simulink model "sgMdl_Serial_RS485Loopback"  (R2024b)
settings: Solver=FixedStepAuto  StartTime=0.0  StopTime=inf  RelTol=1e-3  EnableMultiTasking=on
undefined symbols (not defined in the file): standard
libraries: slrealtimeseriallib x16, speedgoatlib_serial x9
Description:
  | Serial - RS485 Loopback
settings Model: ModifiedByFormat=Speedgoat  Creator=Speedgoat  LastModifiedBy=Speedgoat
settings SolverCC: ConcurrentTasks=on  AlgebraicLoopSolver=TrustRegion  PositivePriorityOrder=on  InsertRTBMode=Never (minimum delay)
settings DataIOCC: LimitDataPoints=on  SaveFormat=Array  SignalLoggingSaveFormat=ModelDataLogs  ReturnWorkspaceOutputs=off
settings OptimizationCC: BlockReduction=off  OptimizeBlockIOStorage=off  BufferReuse=off  GlobalBufferReuse=off  ExpressionFolding=off  ExpressionDepthLimit=2147483647  LocalBlockOutputs=off  OptimizeDataStoreBuffers=off  BusAssignmentInplaceUpdate=off
settings DebuggingCC: UnderspecifiedInitializationDetection=Classic  MergeDetectMultiDrivingBlocksExec=none  SolverPrmCheckMsg=warning  TasksWithSamePriorityMsg=none  FcnCallInpInsideContextMsg=warning  StateNameClashWarn=warning  SFUnexpectedBacktrackingDiag=warning  SFNoUnconditionalDefaultTransitionDiag=warning  SFExecutionAtInitializationDiag=none  ArithmeticOperatorsInVariantConditions=warning
settings HardwareCC: ProdBitPerLong=64  ProdLongLongMode=on  ProdHWDeviceType=Intel->x86-64 (Linux 64)
settings ModelReferenceCC: EnableRefExpFcnMdlSchedulingChecks=on  PropagateSignalLabelsOutOfModel=off
settings SFSimCC: SimUseLocalCustomCode=off  CustomCodeUndefinedFunction=UseInterfaceOnly
settings RTWCC: Description=Speedgoat Real-Time Target Machine  SystemTargetFile=speedgoat.tlc  TemplateMakefile=slrealtime_default_tmf  RTWUseLocalCustomCode=off  Toolchain=Simulink Real-Time Toolchain  BuildConfiguration=Faster Runs  TargetLang=C++  GPUComputeCapability=3.5  DLArmComputeVersion=19.05
settings CodeAppCC: StateflowObjectComments=on
settings SimulinkRealTimeTargetCC: SubcomponentCodeInterfacePackaging=Reusable function  InstructionSetFMA=off  LogToMDFFile=off  SLRTFileLogMaxRuns=10  UseGCCFastMath=on
settings ConfigComp: CovMetricSettings=dw  CovSaveCumulativeToWorkspaceVar=on  CovSaveSingleToWorkspaceVar=on  CovExternalEMLEnable=off  CovSFcnEnable=off  CovBoundaryAbsTol=1.0e-5

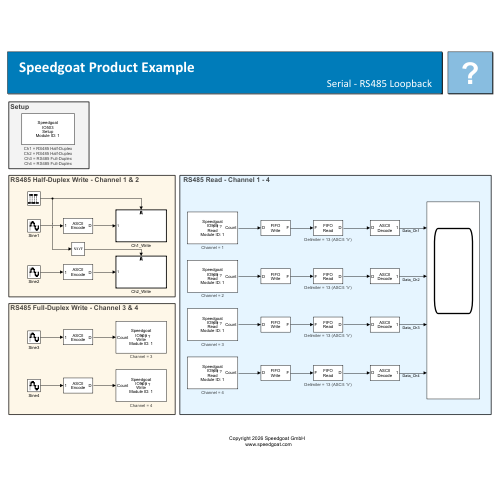
[thumbnail: Simulink's stored preview of the top-level diagram]
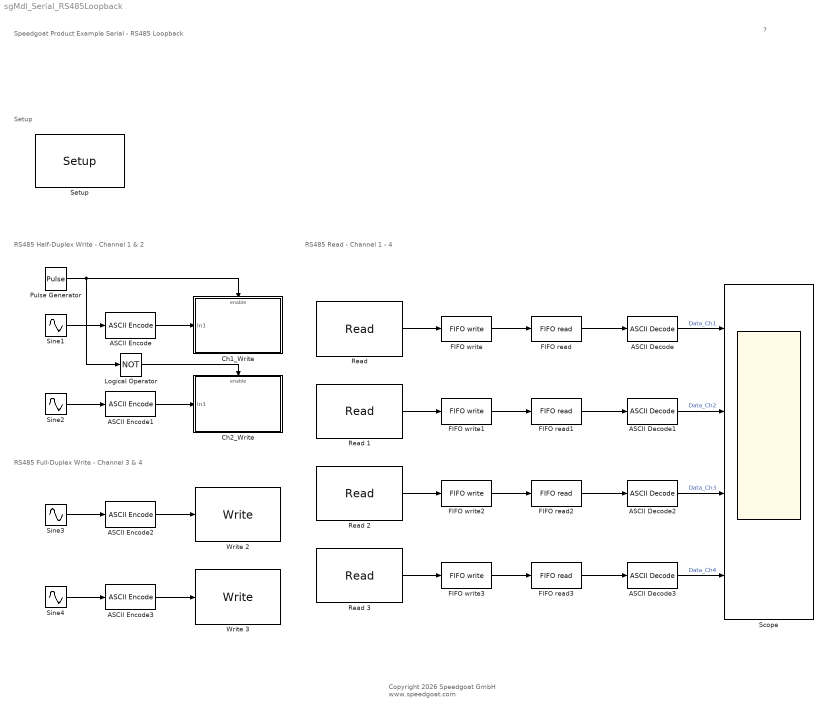
== system sgMdl_Serial_RS485Loopback ==
  note: RS485 Read - Channel 1 - 4
  note: RS485 Half-Duplex Write - Channel 1 & 2
  note: Setup
  note: RS485 Full-Duplex Write - Channel 3 & 4
  note: Speedgoat Product Example
      | Serial - RS485 Loopback
  note: ?
  note: Copyright 2026 Speedgoat GmbH
      |  www.speedgoat.com
  ASCII Decode{,1..3} (4 alike) : slrealtimeseriallib/ASCII Decode  format=%f\r  nvars=1  vartypes={'double'}
  ASCII Encode{,1..3} (4 alike) : slrealtimeseriallib/ASCII Encode  format=%f\r  nvars=1  maxlength=64  vartypes={ 'double' }
  Ch1_Write : Subsystem  TreatAsAtomicUnit=on
  Ch2_Write : Subsystem  TreatAsAtomicUnit=on
  FIFO read{,1..3} (4 alike) : slrealtimeseriallib/FIFO read  maxsize=128  minsize=1  usedelimiter=on  delimiter=13  outputtype=8 bit uint null terminated  enable=off  enableout=off  sampletime=0.01
      settings: AttributesFormatString=Delimiter = %<delimiter> (ASCII: '\r')
  FIFO write : slrealtimeseriallib/FIFO write  size=128  inputtype=8 bit uint null terminated  present=off  sampletime=-1  id=Rx Ch1 overflow
  FIFO write1 : slrealtimeseriallib/FIFO write  size=128  inputtype=8 bit uint null terminated  present=off  sampletime=-1  id=Rx Ch2 overflow
  FIFO write2 : slrealtimeseriallib/FIFO write  size=128  inputtype=8 bit uint null terminated  present=off  sampletime=-1  id=Rx Ch3 overflow
  FIFO write3 : slrealtimeseriallib/FIFO write  size=128  inputtype=8 bit uint null terminated  present=off  sampletime=-1  id=Rx Ch4 overflow
  Logical Operator : Logic  Operator=NOT  AllPortsSameDT=off  OutDataTypeStr=boolean
  Pulse Generator : DiscretePulseGenerator  SampleTime=0.01
  "Read " : speedgoatlib_serial/Speedgoat Shared blocks/Read   parModuleType=IO503  parModuleId=1  parChannel=1  parSampleTime=0.01  parFlush=on  parEnLegacy=on  parDataType=8 bit uint null terminated  parSlot=-1  parRxSwFifoSize=64
      settings: AttributesFormatString=Channel = %<parChannel>
  Read 1 : speedgoatlib_serial/Speedgoat Shared blocks/Read   parModuleType=IO503  parModuleId=1  parChannel=2  parSampleTime=0.01  parFlush=on  parEnLegacy=on  parDataType=8 bit uint null terminated  parSlot=-1  parRxSwFifoSize=64
      settings: AttributesFormatString=Channel = %<parChannel>
  Read 2 : speedgoatlib_serial/Speedgoat Shared blocks/Read   parModuleType=IO503  parModuleId=1  parChannel=3  parSampleTime=0.01  parFlush=on  parEnLegacy=on  parDataType=8 bit uint null terminated  parSlot=-1  parRxSwFifoSize=64
      settings: AttributesFormatString=Channel = %<parChannel>
  Read 3 : speedgoatlib_serial/Speedgoat Shared blocks/Read   parModuleType=IO503  parModuleId=1  parChannel=4  parSampleTime=0.01  parFlush=on  parEnLegacy=on  parDataType=8 bit uint null terminated  parSlot=-1  parRxSwFifoSize=64
      settings: AttributesFormatString=Channel = %<parChannel>
  Scope : Scope  NumInputPorts=4
  "Setup " : speedgoatlib_serial/Speedgoat Shared blocks/Setup   parModuleType=IO503  parModuleId=1  parSlot=-1  parOscillator=44.2368  parOscillator581=125  parTransceiver1=RS485 Half-Duplex  parTransceiver2=RS485 Half-Duplex  parTransceiver3=RS485 Full-Duplex  parTransceiver4=RS485 Full-Duplex  parTransceiver5=Disabled  parTransceiver6=Disabled  parTransceiver7=Disabled  parTransceiver8=Disabled  parTxTerm1=on  parRxTerm1=off  parMessageMonitoring1=off  parAutoTurnaround1=off  parTurnaroundDelay1=0  parStandardBaud1=on  parBaudrate1=2764800  parBaudDivisor1=1  parSamplingRate1=16x (standard)  parPrescale1=None  parCalcBaud1=2764800  parParity1=None  parDataBits1=8  parStopBits1=1  parTxTrigLvl1=1  parRxTrigLvl1=8  parHandshake1=none  parRtsHysteresis1=0  parXon1=17  parXoff1=19  parTxSwFifoSize1=64  parRxSwFifoSize1=64  parTxTerm2=on  parRxTerm2=off  parMessageMonitoring2=off  parAutoTurnaround2=off  parTurnaroundDelay2=0  parStandardBaud2=on  parBaudrate2=2764800  parBaudDivisor2=1  parSamplingRate2=16x (standard)  parPrescale2=None  parCalcBaud2=2764800  parParity2=None  parDataBits2=8  parStopBits2=1  parTxTrigLvl2=1  parRxTrigLvl2=8  parHandshake2=none  parRtsHysteresis2=0  parXon2=17  parXoff2=19  parTxSwFifoSize2=64  parRxSwFifoSize2=64  parTxTerm3=on  parRxTerm3=on  parMessageMonitoring3=off  parAutoTurnaround3=off  parTurnaroundDelay3=0  parStandardBaud3=on  parBaudrate3=2764800  parBaudDivisor3=1  parSamplingRate3=16x (standard)  parPrescale3=None  parCalcBaud3=2764800  parParity3=None  parDataBits3=8  parStopBits3=1  parTxTrigLvl3=1  parRxTrigLvl3=8  parHandshake3=none  parRtsHysteresis3=0  parXon3=17  parXoff3=19  parTxSwFifoSize3=64  parRxSwFifoSize3=64  parTxTerm4=on  parRxTerm4=on  parMessageMonitoring4=off  parAutoTurnaround4=off  parTurnaroundDelay4=0  parStandardBaud4=on  parBaudrate4=2764800  parBaudDivisor4=1  parSamplingRate4=16x (standard)  parPrescale4=None  parCalcBaud4=2764800  parParity4=None  parDataBits4=8  parStopBits4=1  parTxTrigLvl4=1  parRxTrigLvl4=8  parHandshake4=none  parRtsHysteresis4=0  parXon4=17  parXoff4=19  parTxSwFifoSize4=64  parRxSwFifoSize4=64  parTxTerm5=off  parRxTerm5=off  parMessageMonitoring5=off  parAutoTurnaround5=off  parTurnaroundDelay5=0  parStandardBaud5=on  parBaudrate5=115200  parBaudDivisor5=1  parSamplingRate5=16x (standard)  parPrescale5=None  parCalcBaud5=2764800  parParity5=None  parDataBits5=8  parStopBits5=1  parTxTrigLvl5=1  parRxTrigLvl5=1  parHandshake5=none  parRtsHysteresis5=0  parXon5=17  parXoff5=19  parTxSwFifoSize5=1024  parRxSwFifoSize5=1024  parTxTerm6=off  parRxTerm6=off  parMessageMonitoring6=off  parAutoTurnaround6=off  parTurnaroundDelay6=0  parStandardBaud6=on  parBaudrate6=115200  parBaudDivisor6=1  parSamplingRate6=16x (standard)  parPrescale6=None  parCalcBaud6=2764800  parParity6=None  parDataBits6=8  parStopBits6=1  parTxTrigLvl6=1  parRxTrigLvl6=1  parHandshake6=none  parRtsHysteresis6=0  parXon6=17  parXoff6=19  parTxSwFifoSize6=1024  parRxSwFifoSize6=1024  parTxTerm7=off  parRxTerm7=off  parMessageMonitoring7=off  parAutoTurnaround7=off  parTurnaroundDelay7=0  parStandardBaud7=on  parBaudrate7=115200  parBaudDivisor7=1  parSamplingRate7=16x (standard)  parPrescale7=None  parCalcBaud7=2764800  parParity7=None  parDataBits7=8  parStopBits7=1  parTxTrigLvl7=1  parRxTrigLvl7=1  parHandshake7=none  parRtsHysteresis7=0  parXon7=17  parXoff7=19  parTxSwFifoSize7=1024  parRxSwFifoSize7=1024  parTxTerm8=off  parRxTerm8=off  parMessageMonitoring8=off  parAutoTurnaround8=off  parTurnaroundDelay8=0  parStandardBaud8=on  parBaudrate8=115200  parBaudDivisor8=1  parSamplingRate8=16x (standard)  parPrescale8=None  parCalcBaud8=2764800  parParity8=None  parDataBits8=8  parStopBits8=1  parTxTrigLvl8=1  parRxTrigLvl8=1  parHandshake8=none  parRtsHysteresis8=0  parXon8=17  parXoff8=19  parTxSwFifoSize8=1024  parRxSwFifoSize8=1024
      settings: SourceProductName=Simulink Real-Time: Speedgoat I/O Driver Library
      settings: AttributesFormatString=|
      | Ch1 = %<parTransceiver1>
      | Ch2 = %<parTransceiver2>
      | Ch3 = %<parTransceiver3>
      | Ch4 = %<parTransceiver4>
  Sine1 : Sin  Amplitude=10  Bias=127  Frequency=1*2*pi  SampleTime=0.01
  Sine2 : Sin  Amplitude=20  Bias=127  Frequency=1*2*pi  SampleTime=0.01
  Sine3 : Sin  Amplitude=30  Bias=127  Frequency=1*2*pi  SampleTime=0.01
  Sine4 : Sin  Amplitude=40  Bias=127  Frequency=1*2*pi  SampleTime=0.01
  Write 2 : speedgoatlib_serial/Speedgoat Shared blocks/Write   parModuleType=IO503  parModuleId=1  parChannel=3  parSampleTime=-1  parEnLegacy=on  parDataType=8 bit uint null terminated  parMdlStopMsgEnable=off  parMdlStopMsgData=['CONF' char(13)]  parMdlStopFifoOptions=Write to TX FIFO directly  parMdlStopMsgsDataArr=[67 79 78 70 13]  parMdlStopMsgsDataSize=5  parSlot=-1  parTxSwFifoSize=64
      settings: AttributesFormatString=Channel = %<parChannel>
  Write 3 : speedgoatlib_serial/Speedgoat Shared blocks/Write   parModuleType=IO503  parModuleId=1  parChannel=4  parSampleTime=-1  parEnLegacy=on  parDataType=8 bit uint null terminated  parMdlStopMsgEnable=off  parMdlStopMsgData=['CONF' char(13)]  parMdlStopFifoOptions=Write to TX FIFO directly  parMdlStopMsgsDataArr=[67 79 78 70 13]  parMdlStopMsgsDataSize=5  parSlot=-1  parTxSwFifoSize=64
      settings: AttributesFormatString=Channel = %<parChannel>
  wires:
  Sine4/1 -> ASCII Encode3/1
  Sine3/1 -> ASCII Encode2/1
  ASCII Decode/1 -> Scope/1  "Data_Ch1"
  ASCII Decode1/1 -> Scope/2  "Data_Ch2"
  ASCII Decode2/1 -> Scope/3  "Data_Ch3"
  ASCII Decode3/1 -> Scope/4  "Data_Ch4"
  FIFO write/1 -> FIFO read/1
  "Read "/1 -> FIFO write/1
  FIFO write1/1 -> FIFO read1/1
  Read 1/1 -> FIFO write1/1
  FIFO write2/1 -> FIFO read2/1
  FIFO write3/1 -> FIFO read3/1
  FIFO read1/1 -> ASCII Decode1/1
  FIFO read2/1 -> ASCII Decode2/1
  FIFO read3/1 -> ASCII Decode3/1
  Read 2/1 -> FIFO write2/1
  Read 3/1 -> FIFO write3/1
  FIFO read/1 -> ASCII Decode/1
  ASCII Encode2/1 -> Write 2/1
  ASCII Encode3/1 -> Write 3/1
  Pulse Generator/1 -> Ch1_Write/Enable, Logical Operator/1
  Logical Operator/1 -> Ch2_Write/Enable
  Sine1/1 -> ASCII Encode/1
  ASCII Encode/1 -> Ch1_Write/1(In1)
  Sine2/1 -> ASCII Encode1/1
  ASCII Encode1/1 -> Ch2_Write/1(In1)

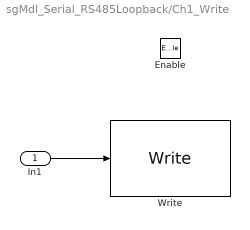
== system sgMdl_Serial_RS485Loopback/Ch1_Write ==
  In1 : Inport
  Enable : EnablePort
  "Write " : speedgoatlib_serial/Speedgoat Shared blocks/Write   parModuleType=IO503  parModuleId=1  parChannel=1  parSampleTime=-1  parEnLegacy=on  parDataType=8 bit uint null terminated  parMdlStopMsgEnable=off  parMdlStopMsgData=['CONF' char(13)]  parMdlStopFifoOptions=Write to TX FIFO directly  parMdlStopMsgsDataArr=[67 79 78 70 13]  parMdlStopMsgsDataSize=5  parSlot=-1  parTxSwFifoSize=64
      settings: AttributesFormatString=Channel = %<parChannel>
  wires:
  In1/1 -> "Write "/1

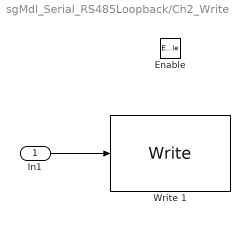
== system sgMdl_Serial_RS485Loopback/Ch2_Write ==
  In1 : Inport
  Enable : EnablePort
  Write 1 : speedgoatlib_serial/Speedgoat Shared blocks/Write   parModuleType=IO503  parModuleId=1  parChannel=2  parSampleTime=-1  parEnLegacy=on  parDataType=8 bit uint null terminated  parMdlStopMsgEnable=off  parMdlStopMsgData=['CONF' char(13)]  parMdlStopFifoOptions=Write to TX FIFO directly  parMdlStopMsgsDataArr=[67 79 78 70 13]  parMdlStopMsgsDataSize=5  parSlot=-1  parTxSwFifoSize=64
      settings: AttributesFormatString=Channel = %<parChannel>
  wires:
  In1/1 -> Write 1/1
